simulink library "Autonomous_lib"  (R2023b)
settings: Solver=VariableStepAuto  StartTime=0.0  StopTime=10.0  RelTol=1e-3
settings Model: Creator=FIRSTMentor  LastModifiedBy=ander

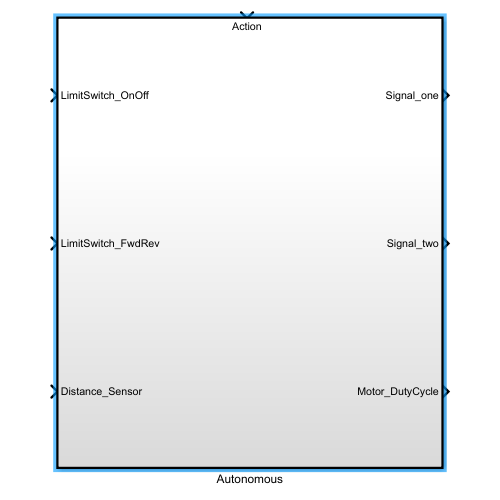
[thumbnail: Simulink's stored preview of the top-level diagram]
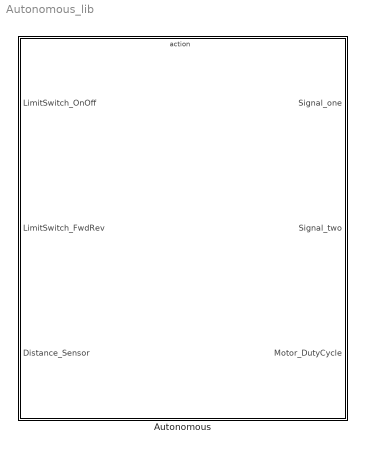
== system Autonomous_lib ==
  Autonomous : Subsystem  TreatAsAtomicUnit=on

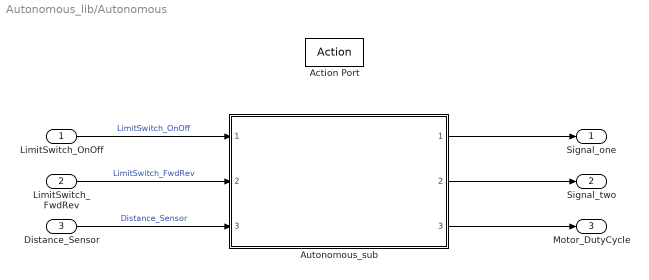
== system Autonomous_lib/Autonomous ==
  LimitSwitch_OnOff : Inport
  LimitSwitch_FwdRev : Inport  Port=2
  Distance_Sensor : Inport  Port=3
  Action Port : ActionPort  InitializeStates=reset
  Autonomous_sub : Subsystem  ReferencedSubsystem=Autonomous_sub
  Signal_one : Outport
  Signal_two : Outport  Port=2
  Motor_DutyCycle : Outport  Port=3
  wires:
  Autonomous_sub/3 -> Motor_DutyCycle/1
  Distance_Sensor/1 -> Autonomous_sub/3  "Distance_Sensor"
  LimitSwitch_FwdRev/1 -> Autonomous_sub/2  "LimitSwitch_FwdRev"
  LimitSwitch_OnOff/1 -> Autonomous_sub/1  "LimitSwitch_OnOff"
  Autonomous_sub/1 -> Signal_one/1
  Autonomous_sub/2 -> Signal_two/1
